simulink model "sim"  (R2024b)
settings: Solver=ode45  StartTime=0.0  StopTime=50  MinStep=0.001  RelTol=1e-3
InitFcn:
  | main
values from neighbouring files (symbols this model uses):
  delta_est = 1/sqrt(2)    [Init.m]    (also in code.m; main.m)
  Kd = Kp * Td    [Init.m]    (also in code.m; main.m)
  Ki = Kp / Ti    [Init.m]    (also in code.m; main.m)
  Kp = deltak * cos(deltaphi)    [Init.m]    (also in code.m = deltak*cos(deltaphi); main.m = deltak*cos(deltaphi))
  pulse2deg = 360/ppr    (= 0.18)    [code.m]    (also in data.m)
  rads2rpm = 60/2/pi    (= 9.54929658551)    [Init.m]    (also in ModelParams.m; data.m; load_params_inertial_case.m)
  tl = 1/(3*wgc)    [Init.m]    (also in code.m = 1/cut_off; main.m = 1/cut_off)
  Ts = 0.001    [Init.m]    (also in ModelParams.m; load_params_inertial_case.m)
  wc = 2*pi*20    (= 125.663706144)    [Init.m]    (also in code.m; main.m)
undefined symbols (not defined in the file or in its folder): daq, drv, gbox, mld, mot, sens, sigbuilder_block
settings Model: Creator=riccardo  LastModifiedBy=Banaan
settings SolverCC: ZeroCrossAlgorithm=Adaptive  AlgebraicLoopSolver=TrustRegion
settings DebuggingCC: IgnoredZcDiagnostic=none  UnconnectedInputMsg=warning  UnconnectedOutputMsg=warning  UnconnectedLineMsg=warning
settings ModelReferenceCC: EnableRefExpFcnMdlSchedulingChecks=on
settings RTWCC: GPUComputeCapability=3.5

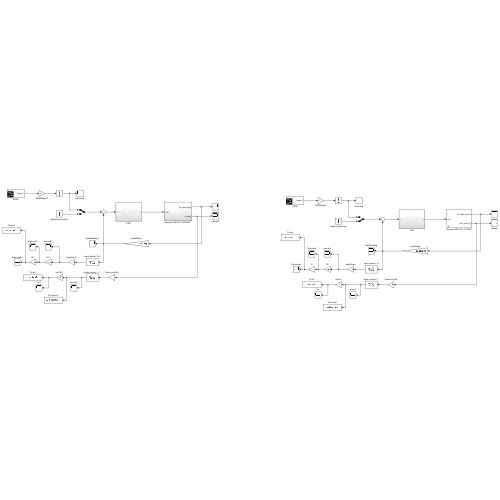
[thumbnail: Simulink's stored preview of the top-level diagram]
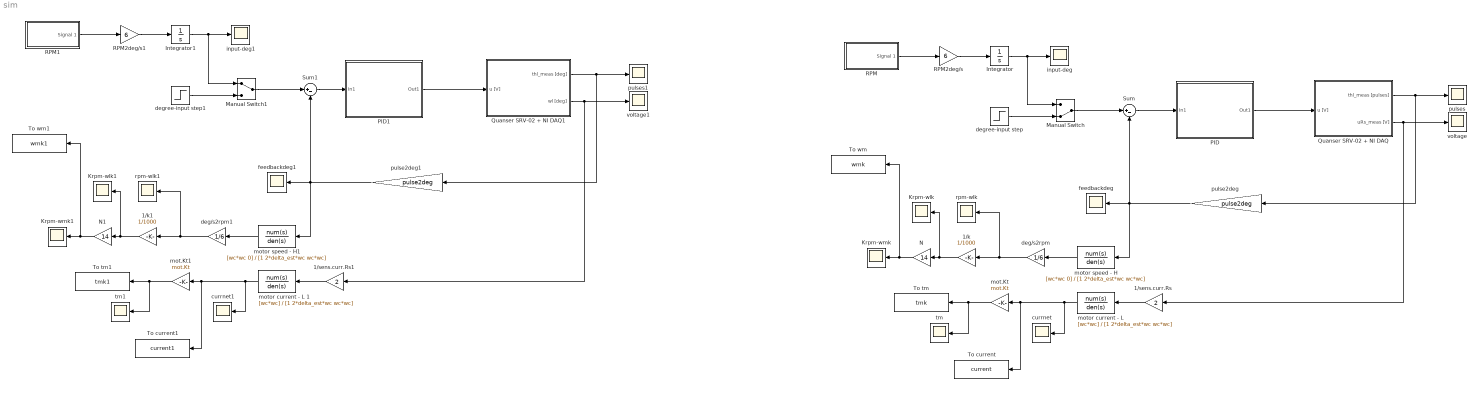
== system sim ==
  1/k : Gain  Gain=1/1000
  1/k1 : Gain  Gain=1/1000
  1/sens.curr.Rs : Gain  Gain=2
  1/sens.curr.Rs1 : Gain  Gain=2
  Integrator : Integrator
  Integrator1 : Integrator
  Krpm-wlk : Scope
  Krpm-wlk1 : Scope
  Krpm-wmk : Scope
  Krpm-wmk1 : Scope
  Manual Switch : ManualSwitch  CurrentSetting=0
  Manual Switch1 : ManualSwitch
  N : Gain  Gain=14
  N1 : Gain  Gain=14
  PID : Subsystem
  PID1 : Subsystem
  Quanser SRV-02 + NI DAQ : Subsystem  mask(Quanser SRV-02 (with inertial load) + NI DAQ){Ts=0.001, fricType=Coulomb + viscous}
      mask prompts: Ts "NI DAQ Sample Time:"; fricType "Friction model"
      mask help: Quanser SRV-02 (with inertial load) + NI DAQ model.
      mask init:
      | %%  Sensors data
      | 
      | %   shunt resistor
      | sens.curr.Rs = 0.5;                         %   resistance [Ohm]   
      | sens.curr.uRs_std = 0.01;                   %   voltage noise standard dev [V]                           
      | sens.curr.uRs_var = sens.curr.uRs_std^2;	%   voltage noise variance [V^2]
      | 
      | %   Hewlett-Packard HEDS-5540#A06 optical encoder
      | sens.enc.ppr = 500*4;                       %   pulses per rotation
      | sens.enc.pulse2deg = 360/sens.enc.ppr;      %   [pulses] -> [deg]
      | sens.enc.pulse2rad = 2*pi/sens.enc.ppr;     %   [pulses] -> [rad]
      | sens.enc.deg2pulse = sens.enc.ppr/360;      %   [deg] -> [pulses]
      | sens.enc.rad2pulse = sens.enc.ppr/2/pi;     %   [rad] -> [pulses]
      | 
      | 
      | %%  Data acquisition board (daq) data
      | 
      | %   NI PCI-6221 DAC data
      | daq.dac.bits = 16;                                  %   resolution (bits)
      | daq.dac.fs   = 10;                                  %   full scale 
      | daq.dac.q    = 2*daq.dac.fs/(2^daq.dac.bits-1);     %	quantization
      | 
      | %   NI PCI-6221 ADC data
      | daq.adc.bits = 16;                                  %   resolution (bits)
      | daq.adc.fs   = 10;                                  %   full scale (as set in SLDRT Analog Input block)
      | daq.adc.q    = 2*daq.adc.fs/(2^daq.adc.bits-1);     %   quantization
      mask Help:
      | Riccardo Antonello (antonello@dei.unipd.it)
      | 
      | April 24, 2020
      | 
      | Dept. of Information Engineering, University of Padova
      mask TypeOptions fricType: Coulomb + viscous | Karnopp
  Quanser SRV-02 + NI DAQ1 : Subsystem
  RPM : Subsystem  Tag=STV Subsys  LoadFcn=sigbuilder_block('load');  StartFcn=sigbuilder_block('start');  StopFcn=sigbuilder_block('stop');  ClipboardFcn=sigbuilder_block('clipboard');  mask(Sigbuilder block){tuvar=[0:10]}
      mask help: Simulink:masks:SigbuilderBlock_MD
      mask init:
      | if ~strcmp(get_param(bdroot(gcbh),'SimulationStatus'),'stopped') tuvar = sigbuilder_block('maskInit'); end
      settings: CopyFcn=sigbuilder_block('copy');  DeleteFcn=sigbuilder_block('delete');  ModelCloseFcn=sigbuilder_block('modelClose');  PreSaveFcn=sigbuilder_block('preSave');  PauseFcn=sigbuilder_block('pause');  ContinueFcn=sigbuilder_block('continue');  NameChangeFcn=sigbuilder_block('namechange');  OpenFcn=sigbuilder_block('open',[4.8 30 1142.4 531.6 ]);  CloseFcn=sigbuilder_block('close');
      mask Display: plot(0, 0, 100, 100,[2, 2, 32, 32, 2], [68, 8, 8, 68, 68],[32, 2], [38, 38], [32, 19, 2],[53, 60, 44], [32, 17, 17, 2],[16, 16, 31, 31]);txt = getActiveGroup(gcbh);text(2, 100, txt,'verticalAlignment', 'top');
  RPM1 : Subsystem  Tag=STV Subsys  LoadFcn=sigbuilder_block('load');  StartFcn=sigbuilder_block('start');  StopFcn=sigbuilder_block('stop');  ClipboardFcn=sigbuilder_block('clipboard');  mask(Sigbuilder block){tuvar=[0:10]}
      mask help: Simulink:masks:SigbuilderBlock_MD
      mask init:
      | if ~strcmp(get_param(bdroot(gcbh),'SimulationStatus'),'stopped') tuvar = sigbuilder_block('maskInit'); end
      settings: CopyFcn=sigbuilder_block('copy');  DeleteFcn=sigbuilder_block('delete');  ModelCloseFcn=sigbuilder_block('modelClose');  PreSaveFcn=sigbuilder_block('preSave');  PauseFcn=sigbuilder_block('pause');  ContinueFcn=sigbuilder_block('continue');  NameChangeFcn=sigbuilder_block('namechange');  OpenFcn=sigbuilder_block('open',[4.8 30 1142.4 531.6 ]);  CloseFcn=sigbuilder_block('close');
      mask Display: plot(0, 0, 100, 100,[2, 2, 32, 32, 2], [68, 8, 8, 68, 68],[32, 2], [38, 38], [32, 19, 2],[53, 60, 44], [32, 17, 17, 2],[16, 16, 31, 31]);txt = getActiveGroup(gcbh);text(2, 100, txt,'verticalAlignment', 'top');
  RPM2deg/s : Gain  Gain=6
  RPM2deg/s1 : Gain  Gain=6
  Sum : Sum  Inputs=|+-
  Sum1 : Sum  Inputs=|+-
  To current : ToWorkspace  VariableName=current  SaveFormat=Timeseries  SampleTime=-1
  To current1 : ToWorkspace  VariableName=current1  SaveFormat=Timeseries  SampleTime=-1
  To tm : ToWorkspace  VariableName=tmk  SaveFormat=Timeseries  SampleTime=-1
  To tm1 : ToWorkspace  VariableName=tmk1  SaveFormat=Timeseries  SampleTime=-1
  To wm : ToWorkspace  VariableName=wmk  SaveFormat=Timeseries  SampleTime=-1
  To wm1 : ToWorkspace  VariableName=wmk1  SaveFormat=Timeseries  SampleTime=-1
  currnet : Scope
  currnet1 : Scope
  deg/s2rpm : Gain  Gain=1/6
  deg/s2rpm1 : Gain  Gain=1/6
  degree-input step : Step  After=180  SampleTime=0
  degree-input step1 : Step  After=180  SampleTime=0
  feedbackdeg : Scope
  feedbackdeg1 : Scope
  input-deg : Scope
  input-deg1 : Scope
  mot.Kt : Gain  Gain=mot.Kt
  mot.Kt1 : Gain  Gain=mot.Kt
  "motor current - L " : TransferFcn  Numerator=[wc*wc]  Denominator=[1 2*delta_est*wc wc*wc]
  motor current - L 1 : TransferFcn  Numerator=[wc*wc]  Denominator=[1 2*delta_est*wc wc*wc]
  motor speed - H : TransferFcn  Numerator=[wc*wc 0]  Denominator=[1 2*delta_est*wc wc*wc]
  motor speed - H1 : TransferFcn  Numerator=[wc*wc 0]  Denominator=[1 2*delta_est*wc wc*wc]
  pulse2deg : Gain  Gain=pulse2deg
  pulse2deg1 : Gain  Gain=pulse2deg
  pulses : Scope
  pulses1 : Scope
  rpm-wlk : Scope
  rpm-wlk1 : Scope
  tm : Scope
  tm1 : Scope
  voltage : Scope
  voltage1 : Scope
  wires:
  Sum/1 -> PID/1(In1)
  PID/1(Out1) -> Quanser SRV-02 + NI DAQ/1(u [V])
  Quanser SRV-02 + NI DAQ/1(thl_meas [pulses]) -> pulses/1, pulse2deg/1
  Quanser SRV-02 + NI DAQ/2(uRs_meas [V]) -> 1/sens.curr.Rs/1, voltage/1
  RPM/1(Signal 1) -> RPM2deg/s/1
  Integrator/1 -> Manual Switch/1, input-deg/1
  RPM2deg/s/1 -> Integrator/1
  pulse2deg/1 -> motor speed - H/1, feedbackdeg/1, Sum/2
  motor speed - H/1 -> deg/s2rpm/1
  deg/s2rpm/1 -> rpm-wlk/1, 1/k/1
  degree-input step/1 -> Manual Switch/2
  Manual Switch/1 -> Sum/1
  1/k/1 -> Krpm-wlk/1, N/1
  N/1 -> To wm/1, Krpm-wmk/1
  "motor current - L "/1 -> mot.Kt/1, To current/1, currnet/1
  1/sens.curr.Rs/1 -> "motor current - L "/1
  mot.Kt/1 -> tm/1, To tm/1
  mot.Kt1/1 -> To tm1/1, tm1/1
  1/sens.curr.Rs1/1 -> motor current - L 1/1
  motor current - L 1/1 -> currnet1/1, To current1/1, mot.Kt1/1
  N1/1 -> Krpm-wmk1/1, To wm1/1
  1/k1/1 -> N1/1, Krpm-wlk1/1
  Manual Switch1/1 -> Sum1/1
  degree-input step1/1 -> Manual Switch1/2
  deg/s2rpm1/1 -> 1/k1/1, rpm-wlk1/1
  motor speed - H1/1 -> deg/s2rpm1/1
  pulse2deg1/1 -> Sum1/2, feedbackdeg1/1, motor speed - H1/1
  RPM2deg/s1/1 -> Integrator1/1
  Integrator1/1 -> input-deg1/1, Manual Switch1/1
  RPM1/1(Signal 1) -> RPM2deg/s1/1
  Quanser SRV-02 + NI DAQ1/2(wl [deg]) -> voltage1/1, 1/sens.curr.Rs1/1
  Quanser SRV-02 + NI DAQ1/1(thl_meas [deg]) -> pulse2deg1/1, pulses1/1
  PID1/1(Out1) -> Quanser SRV-02 + NI DAQ1/1(u [V])
  Sum1/1 -> PID1/1(In1)

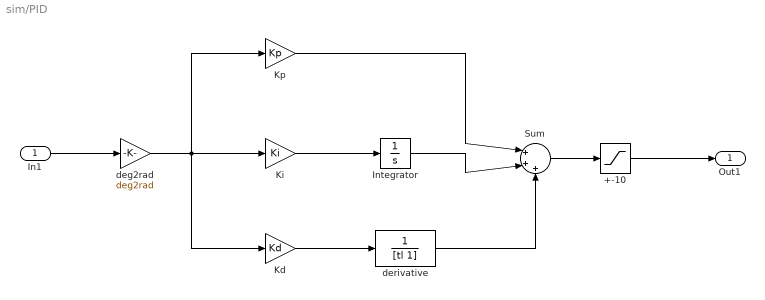
== system sim/PID ==
  In1 : Inport
  +-10 : Saturate  UpperLimit=10  LowerLimit=-10
  Integrator : Integrator
  Kd : Gain  Gain=Kd
  Ki : Gain  Gain=Ki
  Kp : Gain  Gain=Kp
  Sum : Sum  Inputs=|+++
  deg2rad : Gain  Gain=deg2rad
  derivative : TransferFcn  Denominator=[tl 1]
  Out1 : Outport
  wires:
  In1/1 -> deg2rad/1
  deg2rad/1 -> Kd/1, Kp/1, Ki/1
  Ki/1 -> Integrator/1
  Kp/1 -> Sum/1
  Integrator/1 -> Sum/2
  Kd/1 -> derivative/1
  derivative/1 -> Sum/3
  Sum/1 -> +-10/1
  +-10/1 -> Out1/1

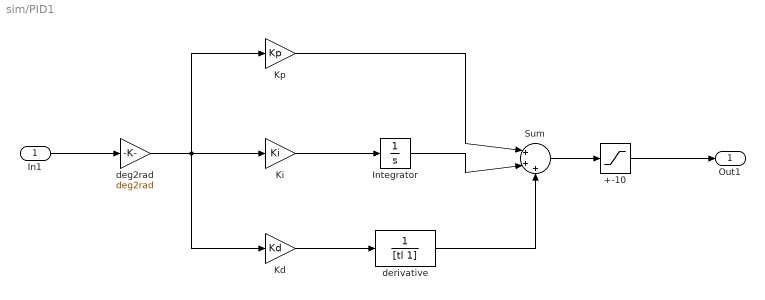
== system sim/PID1 ==
  In1 : Inport
  +-10 : Saturate  UpperLimit=10  LowerLimit=-10
  Integrator : Integrator
  Kd : Gain  Gain=Kd
  Ki : Gain  Gain=Ki
  Kp : Gain  Gain=Kp
  Sum : Sum  Inputs=|+++
  deg2rad : Gain  Gain=deg2rad
  derivative : TransferFcn  Denominator=[tl 1]
  Out1 : Outport
  wires:
  +-10/1 -> Out1/1
  Sum/1 -> +-10/1
  derivative/1 -> Sum/3
  Kd/1 -> derivative/1
  Integrator/1 -> Sum/2
  Kp/1 -> Sum/1
  Ki/1 -> Integrator/1
  deg2rad/1 -> Ki/1, Kp/1, Kd/1
  In1/1 -> deg2rad/1

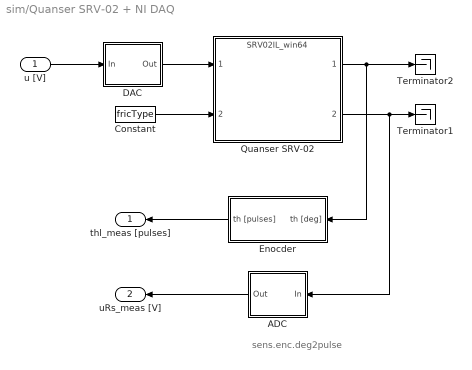
== system sim/Quanser SRV-02 + NI DAQ ==
  note: sens.enc.deg2pulse
  u [V] : Inport
  ADC : Subsystem
  Constant : Constant  Value=fricType
  DAC : Subsystem
  Enocder : Subsystem
  Quanser SRV-02 : ModelReference  ModelNameDialog=SRV02IL_win64.slxp  ModelReferenceVersion=1.44  CopyOfModelProtected=on
  Terminator1 : Terminator
  Terminator2 : Terminator
  thl_meas [pulses] : Outport
  uRs_meas [V] : Outport  Port=2
  wires:
  Enocder/1(th [pulses]) -> thl_meas [pulses]/1
  ADC/1(Out) -> uRs_meas [V]/1
  DAC/1(Out) -> Quanser SRV-02/1
  Quanser SRV-02/2 -> ADC/1(In), Terminator1/1
  u [V]/1 -> DAC/1(In)
  Quanser SRV-02/1 -> Enocder/1(th [deg]), Terminator2/1
  Constant/1 -> Quanser SRV-02/2

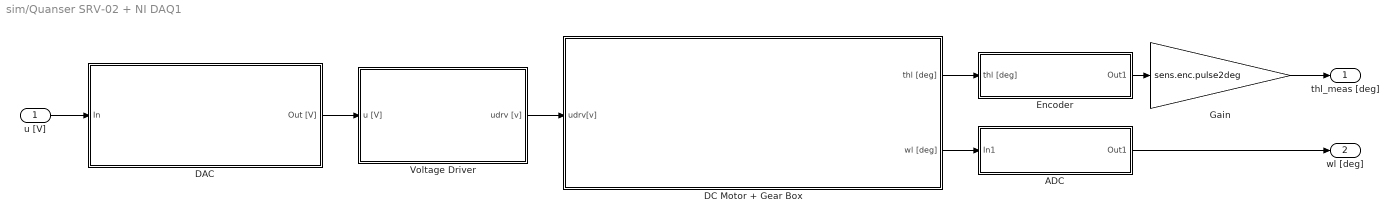
== system sim/Quanser SRV-02 + NI DAQ1 ==
  u [V] : Inport
  ADC : Subsystem
  DAC : Subsystem
  DC Motor + Gear Box : Subsystem
  Encoder : Subsystem
  Gain : Gain  Gain=sens.enc.pulse2deg
  Voltage Driver : Subsystem
  thl_meas [deg] : Outport
  wl [deg] : Outport  Port=2
  wires:
  Gain/1 -> thl_meas [deg]/1
  ADC/1(Out1) -> wl [deg]/1
  DC Motor + Gear Box/1(thl [deg]) -> Encoder/1(thl [deg])
  DC Motor + Gear Box/2(wl [deg]) -> ADC/1(In1)
  Voltage Driver/1(udrv [v]) -> DC Motor + Gear Box/1(udrv[v])
  DAC/1(Out [V]) -> Voltage Driver/1(u [V])
  u [V]/1 -> DAC/1(In)
  Encoder/1(Out1) -> Gain/1

== system sim/RPM ==
  Demux : Demux  Tag=STV Demux  Outputs=1
      settings: DisplayOption=none
  FromWs : FromWorkspace  Tag=STV FromWs  VariableName=tuvar
      SigBuilderData=|
      | common.afterFinalStr = 'Extrapolate'
      | common.sampleTime = 0
      | dataSet.timeRange = [0 45]
      | dataSet.name = 'Group 1'
      | sbobj.Groups.Name = 'Group 1'
      | sbobj.Groups.Signals.Name = 'Signal 1'
      | sbobj.Groups.Signals.XData = [0 5 5 10 10 15 15 20 20 25 25 30 30 35 35 40 40 45]
      | sbobj.Groups.Signals.YData = [50 50 100 100 150 150 200 200 250 250 300 300 350 350 400 400 450 450]
      | sbobj.Groups.TimeRange = [0 45]
  Signal 1 : Outport  Tag=STV Outport
  wires:
  Demux/1 -> Signal 1/1
  FromWs/1 -> Demux/1

== system sim/RPM1 ==
  Demux : Demux  Tag=STV Demux  Outputs=1
      settings: DisplayOption=none
  FromWs : FromWorkspace  Tag=STV FromWs  VariableName=tuvar
      SigBuilderData=|
      | common.afterFinalStr = 'Extrapolate'
      | common.sampleTime = 0
      | dataSet.timeRange = [0 45]
      | dataSet.name = 'Group 1'
      | sbobj.Groups.Name = 'Group 1'
      | sbobj.Groups.Signals.Name = 'Signal 1'
      | sbobj.Groups.Signals.XData = [0 5 5 10 10 15 15 20 20 25 25 30 30 35 35 40 40 45]
      | sbobj.Groups.Signals.YData = [50 50 100 100 150 150 200 200 250 250 300 300 350 350 400 400 450 450]
      | sbobj.Groups.TimeRange = [0 45]
  Signal 1 : Outport  Tag=STV Outport
  wires:
  FromWs/1 -> Demux/1
  Demux/1 -> Signal 1/1

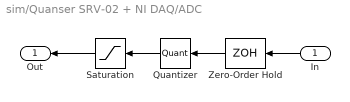
== system sim/Quanser SRV-02 + NI DAQ/ADC ==
  In : Inport
  Quantizer : Quantizer  QuantizationInterval=daq.adc.q
  Saturation : Saturate  UpperLimit=daq.adc.fs  LowerLimit=-daq.adc.fs
  Zero-Order Hold : ZeroOrderHold  SampleTime=Ts
  Out : Outport
  wires:
  Saturation/1 -> Out/1
  In/1 -> Zero-Order Hold/1
  Quantizer/1 -> Saturation/1
  Zero-Order Hold/1 -> Quantizer/1

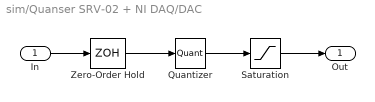
== system sim/Quanser SRV-02 + NI DAQ/DAC ==
  In : Inport
  Quantizer : Quantizer  QuantizationInterval=daq.dac.q
  Saturation : Saturate  UpperLimit=daq.dac.fs  LowerLimit=-daq.dac.fs
  Zero-Order Hold : ZeroOrderHold  SampleTime=Ts
  Out : Outport
  wires:
  Quantizer/1 -> Saturation/1
  In/1 -> Zero-Order Hold/1
  Zero-Order Hold/1 -> Quantizer/1
  Saturation/1 -> Out/1

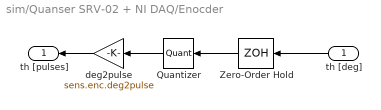
== system sim/Quanser SRV-02 + NI DAQ/Enocder ==
  th [deg] : Inport
  Quantizer : Quantizer  QuantizationInterval=sens.enc.pulse2deg
  Zero-Order Hold : ZeroOrderHold  SampleTime=Ts
  deg2pulse : Gain  Gain=sens.enc.deg2pulse
  th [pulses] : Outport
  wires:
  Quantizer/1 -> deg2pulse/1
  th [deg]/1 -> Zero-Order Hold/1
  Zero-Order Hold/1 -> Quantizer/1
  deg2pulse/1 -> th [pulses]/1

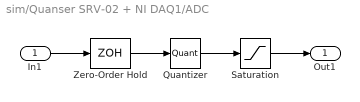
== system sim/Quanser SRV-02 + NI DAQ1/ADC ==
  In1 : Inport
  Quantizer : Quantizer  QuantizationInterval=daq.adc.q
  Saturation : Saturate  UpperLimit=daq.adc.fs  LowerLimit=-daq.adc.fs
  Zero-Order Hold : ZeroOrderHold  SampleTime=Ts
  Out1 : Outport
  wires:
  Zero-Order Hold/1 -> Quantizer/1
  Quantizer/1 -> Saturation/1
  In1/1 -> Zero-Order Hold/1
  Saturation/1 -> Out1/1

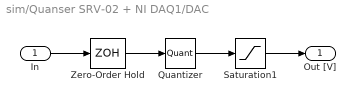
== system sim/Quanser SRV-02 + NI DAQ1/DAC ==
  In : Inport
  Quantizer : Quantizer  QuantizationInterval=daq.adc.q
  Saturation1 : Saturate  UpperLimit=daq.dac.fs  LowerLimit=-daq.dac.fs
  Zero-Order Hold : ZeroOrderHold  SampleTime=Ts
  Out [V] : Outport
  wires:
  Saturation1/1 -> Out [V]/1
  Zero-Order Hold/1 -> Quantizer/1
  Quantizer/1 -> Saturation1/1
  In/1 -> Zero-Order Hold/1

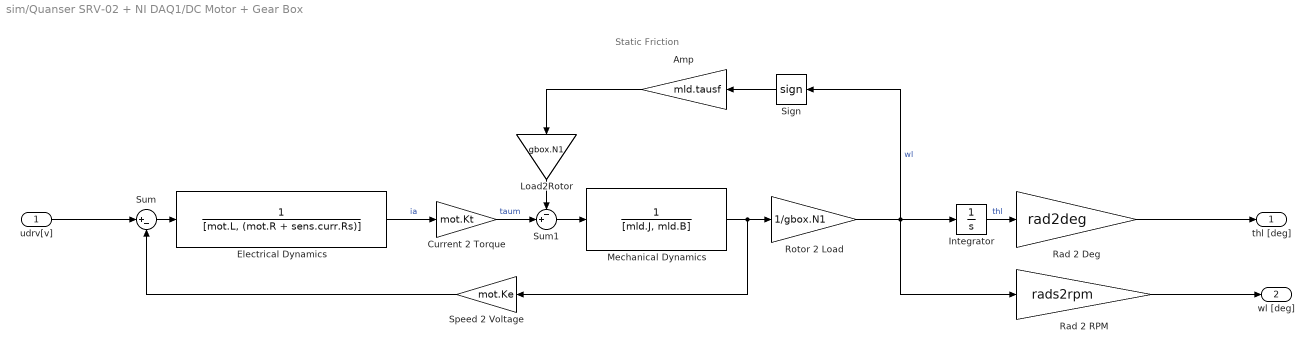
== system sim/Quanser SRV-02 + NI DAQ1/DC Motor + Gear Box ==
  note: Static Friction
  udrv[v] : Inport
  Amp : Gain  Gain=mld.tausf
  Current 2 Torque : Gain  Gain=mot.Kt
  Electrical Dynamics : TransferFcn  Numerator=1  Denominator=[mot.L, (mot.R + sens.curr.Rs)]
  Integrator : Integrator
  Load2Rotor : Gain  Gain=gbox.N1
  Mechanical Dynamics : TransferFcn  Denominator=[mld.J, mld.B]
  Rad 2 Deg : Gain  Gain=rad2deg
  Rad 2 RPM : Gain  Gain=rads2rpm
  Rotor 2 Load : Gain  Gain=1/gbox.N1
  Sign : Signum
  Speed 2 Voltage : Gain  Gain=mot.Ke
  Sum : Sum  Inputs=|+-
  Sum1 : Sum  Inputs=-+|
  thl [deg] : Outport
  wl [deg] : Outport  Port=2
  wires:
  Rad 2 RPM/1 -> wl [deg]/1
  udrv[v]/1 -> Sum/1
  Rad 2 Deg/1 -> thl [deg]/1
  Current 2 Torque/1 -> Sum1/2  "taum"
  Rotor 2 Load/1 -> Sign/1, Integrator/1, Rad 2 RPM/1  "wl"
  Sum1/1 -> Mechanical Dynamics/1
  Electrical Dynamics/1 -> Current 2 Torque/1  "ia"
  Integrator/1 -> Rad 2 Deg/1  "thl"
  Sign/1 -> Amp/1
  Speed 2 Voltage/1 -> Sum/2
  Mechanical Dynamics/1 -> Speed 2 Voltage/1, Rotor 2 Load/1
  Load2Rotor/1 -> Sum1/1
  Amp/1 -> Load2Rotor/1
  Sum/1 -> Electrical Dynamics/1

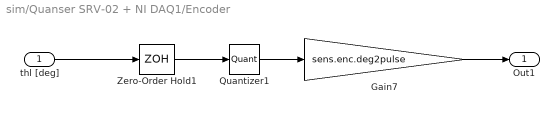
== system sim/Quanser SRV-02 + NI DAQ1/Encoder ==
  thl [deg] : Inport
  Gain7 : Gain  Gain=sens.enc.deg2pulse
  Quantizer1 : Quantizer  QuantizationInterval=sens.enc.pulse2deg
  Zero-Order Hold1 : ZeroOrderHold  SampleTime=Ts
  Out1 : Outport
  wires:
  Quantizer1/1 -> Gain7/1
  thl [deg]/1 -> Zero-Order Hold1/1
  Gain7/1 -> Out1/1
  Zero-Order Hold1/1 -> Quantizer1/1

== system sim/Quanser SRV-02 + NI DAQ1/Voltage Driver ==
  u [V] : Inport
  Saturation : Saturate  UpperLimit=drv.outmax  LowerLimit=-drv.outmax
  Transfer Fcn2 : TransferFcn  Numerator=drv.dcgain  Denominator=[drv.Tc 1]
  udrv [v] : Outport
  wires:
  Saturation/1 -> udrv [v]/1
  Transfer Fcn2/1 -> Saturation/1
  u [V]/1 -> Transfer Fcn2/1
